simulink model "Labormodell_2014"  (R2014b)
settings: Solver=ode45  StartTime=0.0  StopTime=10.0  RelTol=1e-3
undefined symbols (not defined in the file): A_ss, B_ss, C_ss, P_t_0, Q, q_max, q_min, R, v, w
settings Model: CovSFcnEnable=on  Creator=gonzalocastritius  LastModifiedBy=labor09
settings DebuggingCC: UnderspecifiedInitializationDetection=Classic  MergeDetectMultiDrivingBlocksExec=none  FrameProcessingCompatibilityMsg=error  StateNameClashWarn=warning

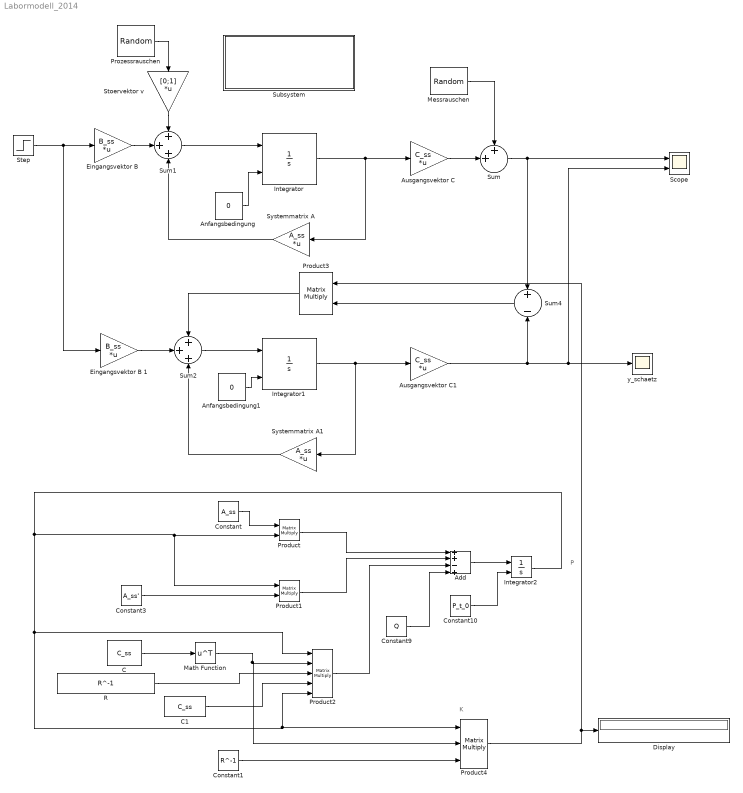
== system Labormodell_2014 ==
  note: K
  note: P
  Add : Sum  Inputs=++-+
  Anfangsbedingung : Constant  Value=0
  Anfangsbedingung1 : Constant  Value=0
  Ausgangsvektor C : Gain  Gain=C_ss  Multiplication=Matrix(K*u)
  Ausgangsvektor C1 : Gain  Gain=C_ss  Multiplication=Matrix(K*u)
  C : Constant  Value=C_ss  VectorParams1D=off
  C1 : Constant  Value=C_ss  VectorParams1D=off
  Constant : Constant  Value=A_ss
  Constant1 : Constant  Value=R^-1
  Constant10 : Constant  Value=P_t_0
  Constant3 : Constant  Value=A_ss'
  Constant9 : Constant  Value=Q  VectorParams1D=off
  Display : Display
  "Eingangsvektor B " : Gain  Gain=B_ss  Multiplication=Matrix(K*u)
  Eingangsvektor B 1 : Gain  Gain=B_ss  Multiplication=Matrix(K*u)
  Integrator : Integrator  InitialConditionSource=external  UpperSaturationLimit=q_max  LowerSaturationLimit=q_min
  Integrator1 : Integrator  InitialConditionSource=external  UpperSaturationLimit=q_max  LowerSaturationLimit=q_min
  Integrator2 : Integrator  InitialConditionSource=external
  Math Function : Math  Operator=transpose  SaturateOnIntegerOverflow=on
  Messrauschen : RandomNumber  Variance=w  SampleTime=0.01
  Product : Product  Multiplication=Matrix(*)
  Product1 : Product  Multiplication=Matrix(*)
  Product2 : Product  Inputs=5  Multiplication=Matrix(*)
  Product3 : Product  Multiplication=Matrix(*)
  Product4 : Product  Inputs=3  Multiplication=Matrix(*)
  Prozessrauschen : RandomNumber  Variance=v  SampleTime=0.01
  R : Constant  Value=R^-1  VectorParams1D=off
  Scope : Scope  NumInputPorts=2
      settings: TimeRange=auto  MaxDataPoints=5000  SaveToWorkspace=off  SaveName=ScopeData  YMin=-3.19306~-1.35412  YMax=13.38703~12.18705  SampleTime=-1
  Step : Step  After=100  SampleTime=0
  Stoervektor v : Gain  Gain=[0;1]  Multiplication=Matrix(K*u)
  Subsystem : Subsystem
      settings: OpenFcn=Parameter_Versuch
      mask Display: fprintf('Doppelklick um Parameter zu laden')
  Sum : Sum  Inputs=++|
  Sum1 : Sum  Inputs=+++
  Sum2 : Sum  Inputs=+++
  Sum4 : Sum  Inputs=+-
  Systemmatrix A : Gain  Gain=A_ss  Multiplication=Matrix(K*u)
  Systemmatrix A1 : Gain  Gain=A_ss  Multiplication=Matrix(K*u)
  y_schaetz : Scope
      settings: TimeRange=auto  MaxDataPoints=5000  SaveToWorkspace=off  YMin=-1.35412  YMax=12.18705  SampleTime=-1
  wires:
  "Eingangsvektor B "/1 -> Sum1/2
  Anfangsbedingung/1 -> Integrator/2
  Ausgangsvektor C/1 -> Sum/2
  Integrator/1 -> Systemmatrix A/1, Ausgangsvektor C/1
  Sum1/1 -> Integrator/1
  Systemmatrix A/1 -> Sum1/3
  Stoervektor v/1 -> Sum1/1
  Messrauschen/1 -> Sum/1
  Prozessrauschen/1 -> Stoervektor v/1
  Sum/1 -> Scope/1, Sum4/1
  Step/1 -> Eingangsvektor B 1/1, "Eingangsvektor B "/1
  Eingangsvektor B 1/1 -> Sum2/2
  Sum2/1 -> Integrator1/1
  Anfangsbedingung1/1 -> Integrator1/2
  Integrator1/1 -> Systemmatrix A1/1, Ausgangsvektor C1/1
  Systemmatrix A1/1 -> Sum2/3
  Product3/1 -> Sum2/1
  Sum4/1 -> Product3/2
  Ausgangsvektor C1/1 -> Scope/2, y_schaetz/1, Sum4/2
  Constant/1 -> Product/1
  Constant3/1 -> Product1/2
  Product/1 -> Add/1
  Product1/1 -> Add/2
  C/1 -> Math Function/1
  Product2/1 -> Add/3
  Constant9/1 -> Add/4
  R/1 -> Product2/3
  C1/1 -> Product2/4
  Integrator2/1 -> Product2/5, Product4/1, Product2/1, Product/2, Product1/1
  Add/1 -> Integrator2/1
  Constant10/1 -> Integrator2/2
  Product4/1 -> Product3/1, Display/1
  Constant1/1 -> Product4/3
  Math Function/1 -> Product4/2, Product2/2

== system Labormodell_2014/Subsystem ==
